simulink model "simulazione_simulink_punto4"  (R2023a)
settings: Solver=VariableStepAuto  StartTime=0.0  StopTime=50  RelTol=1e-3
values from neighbouring files (symbols this model uses):
  A = [0,0,1,0 ; 0,0,0,1 ; -k/m1, k/m1, -c/m1, c/m1 ; k/m2, -k/m2, c/m2, -c/m2]    [Test.m]    (also in Test.mat = [0 0 -0.1 0.133333333333 0 0 0.1 -0.133333333333 1 0 -0.25 0)
  B = [0 ; 0 ; 1/m1 ; 0]    [Test.m]    (also in Test.mat = [0 0 0.0005 0])
  C = [1, 0, 0, 0]    [Test.m]    (also in Test.mat = [1 0 0 0])
  D = 0    [Test.m]
  M = [0 ; 0 ; 0 ; 1/m2]    [Test.m]    (also in Test.mat = [0 0 0 0.000666666666667])
  V = transpose(K)    [Test.m]
undefined symbols (not defined in the file or in its folder): g1, g2, g3, g4, g5, gaussian, L, max_disturbo, min_disturbo, x_0, x_0_stimato
libraries: simulink x1
settings Model: Creator=simon  LastModifiedBy=valeria
settings OptimizationCC: ReuseModelBlockBuffer=off

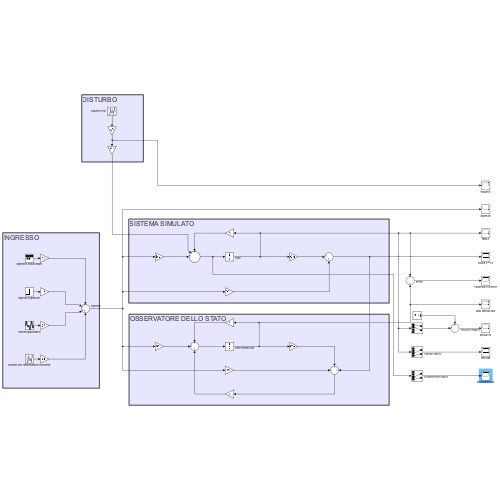
[thumbnail: Simulink's stored preview of the top-level diagram]
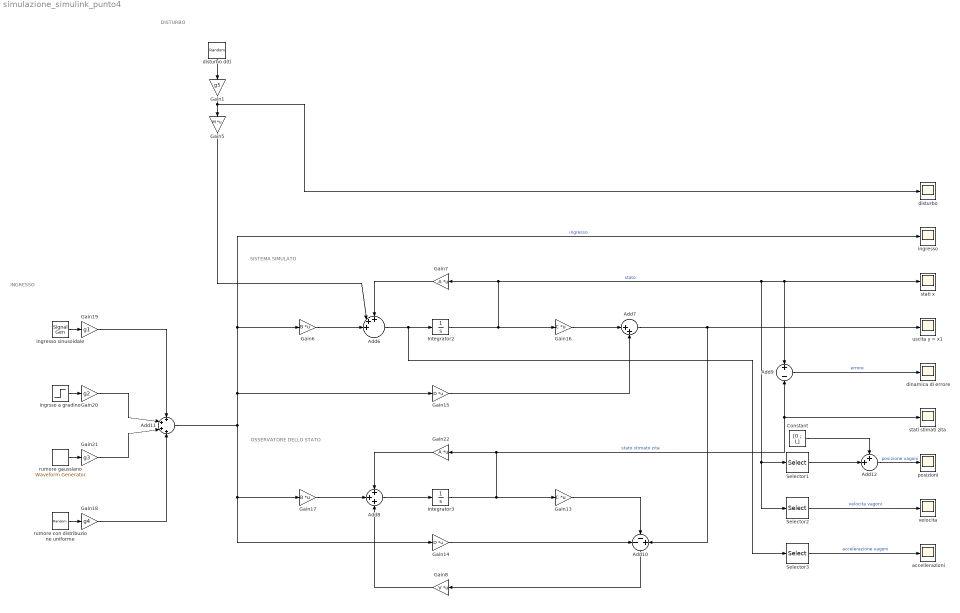
== system simulazione_simulink_punto4 ==
  note: DISTURBO
  note: INGRESSO
  note: SISTEMA SIMULATO
  note: OSSERVATORE DELLO STATO
  Add10 : Sum  Inputs=--+
  Add11 : Sum  Inputs=++++
  Add12 : Sum  Inputs=++|
  Add6 : Sum  Inputs=+++||
  Add7 : Sum  Inputs=|++
  Add8 : Sum  Inputs=+++
  Add9 : Sum  Inputs=+-
  Constant : Constant  Value=[0 ; L]
  Gain1 : Gain  Gain=g5
  Gain13 : Gain  Gain=C  Multiplication=Matrix(K*u)
  Gain14 : Gain  Gain=D  Multiplication=Matrix(K*u)
  Gain15 : Gain  Gain=D  Multiplication=Matrix(K*u)
  Gain16 : Gain  Gain=C  Multiplication=Matrix(K*u)
  Gain17 : Gain  Gain=B  Multiplication=Matrix(K*u)
  Gain18 : Gain  Gain=g4
  Gain19 : Gain  Gain=g1
  Gain20 : Gain  Gain=g2
  Gain21 : Gain  Gain=g3
  Gain22 : Gain  Gain=A  Multiplication=Matrix(K*u)
  Gain5 : Gain  Gain=M  Multiplication=Matrix(K*u)
  Gain6 : Gain  Gain=B  Multiplication=Matrix(K*u)
  Gain7 : Gain  Gain=A  Multiplication=Matrix(K*u)
  Gain8 : Gain  Gain=V  Multiplication=Matrix(K*u)
  Integrator2 : Integrator  InitialCondition=x_0
  Integrator3 : Integrator  InitialCondition=x_0_stimato
  Selector1 : Selector  InputPortWidth=4  IndexOptions=Index vector (dialog)  Indices=[1 2]  OutputSizes=1  RuntimeRangeChecks=on
  Selector2 : Selector  InputPortWidth=4  IndexOptions=Index vector (dialog)  Indices=[3 4]  OutputSizes=1  RuntimeRangeChecks=on
  Selector3 : Selector  InputPortWidth=4  IndexOptions=Index vector (dialog)  Indices=[3 4]  OutputSizes=1  RuntimeRangeChecks=on
  accellerazioni : Scope
  dinamica di errore : Scope
  disturbo : Scope
  disturbo d(t) : UniformRandomNumber  Minimum=min_disturbo  Maximum=max_disturbo  SampleTime=0.1
  ingresso : Scope
  ingresso sinusoidale : SignalGenerator
  ingrsso a gradino : Step  Time=0  SampleTime=0  ZeroCross=off
  posizioni : Scope
  rumore con distribuzione uniforme : UniformRandomNumber  SampleTime=0.1
  rumore gaussiano : simulink/Sources/Waveform Generator  OutMin=[]  OutMax=[]  OutDataTypeStr=double  SelectedSignal=1  Signals=gaussian()  BlockNames=MultiportSwitch_746ec0809bf24cb  SampleTime=0.1
  stati stimati zita : Scope
  stati x : Scope
  uscita y = x1 : Scope
  velocita : Scope
  wires:
  disturbo d(t)/1 -> Gain1/1
  Add9/1 -> dinamica di errore/1  "errore"
  Add10/1 -> Gain8/1
  Constant/1 -> Add12/1
  Gain16/1 -> Add7/1
  Selector2/1 -> velocita/1  "velocita vagoni"
  Add11/1 -> Gain14/1, Gain17/1, Gain15/1, ingresso/1, Gain6/1  "ingresso"
  Gain21/1 -> Add11/3
  Integrator2/1 -> Gain16/1, Selector1/1, Selector2/1, stati x/1, Add9/1, Gain7/1  "stato"
  Add7/1 -> Add10/3, uscita y = x1/1
  ingresso sinusoidale/1 -> Gain19/1
  Gain13/1 -> Add10/2
  Gain17/1 -> Add8/2
  Gain19/1 -> Add11/1
  Integrator3/1 -> Gain22/1, Add9/2, stati stimati zita/1, Gain13/1  "stato stimato zita"
  Gain6/1 -> Add6/3
  Gain14/1 -> Add10/1
  rumore gaussiano/1 -> Gain21/1
  ingrsso a gradino/1 -> Gain20/1
  Gain20/1 -> Add11/2
  Gain15/1 -> Add7/2
  Gain8/1 -> Add8/3
  rumore con distribuzione uniforme/1 -> Gain18/1
  Add6/1 -> Selector3/1, Integrator2/1
  Gain7/1 -> Add6/1
  Gain22/1 -> Add8/1
  Gain18/1 -> Add11/4
  Add8/1 -> Integrator3/1
  Gain1/1 -> Gain5/1, disturbo/1
  Gain5/1 -> Add6/2
  Add12/1 -> posizioni/1  "posizione vagoni"
  Selector1/1 -> Add12/2
  Selector3/1 -> accellerazioni/1  "accelerazione vagoni"
